simulink model "Single_Phase_Rectifier"  (R2023b)
settings: Solver=VariableStepAuto  StartTime=0.0  StopTime=0.1  MaxStep=2e-4  RelTol=1e-3
libraries: spsDetailedThyristorLib x4, spsACVoltageSourceLib x1, spsMultimeterLib x1, spsSeriesRLCBranchLib x1, sps_lib x1
settings Model: Creator=33034  LastModifiedBy=33034

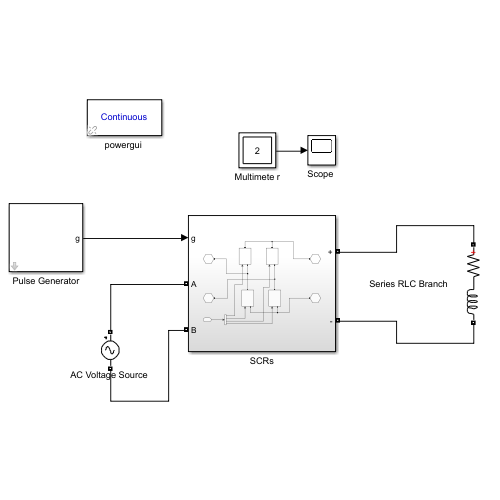
[thumbnail: Simulink's stored preview of the top-level diagram]
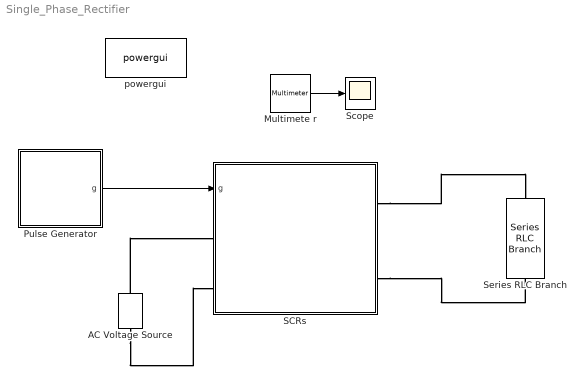
== system Single_Phase_Rectifier ==
  "AC Voltage Source " : spsACVoltageSourceLib/AC Voltage Source  Amplitude=220*sqrt(2)  Phase=0  Frequency=50  SampleTime=0  Measurements=None  BusType=swing  Pref=10e3  Qref=0  Qmin=-inf  Qmax=+inf
  Multimete r : spsMultimeterLib/Multimeter  L=2  sel=[1 2]  yselected={}  Gain=[1 1]  OutputType=Complex  PlotAtSimulationStop=off  PhasorSimulation=off
  Pulse Generator : Subsystem  mask{freq=50, alpha=90}
      mask prompts: freq "频率"
      mask DialogControl ParameterGroupVar Prompt: 参数
  SCRs : Subsystem
  "Scope " : Scope
  "Series RLC Branch " : spsSeriesRLCBranchLib/Series RLC Branch  LConnTagsString=__new0  RConnTagsString=__new0  BranchType=RL  Resistance=10  Inductance=1  SetiL0=off  InitialCurrent=0  Capacitance=1e-6  Setx0=off  InitialVoltage=0  Measurements=Branch voltage and current
  "powergui " : sps_lib/powergui  Priority=1  SimulationMode=Continuous  SampleTime=50e-6  frequency=60  Iterations=50  frequencyindice=50  Pbase=100e6  ErrMax=1e-4  UnitsV=kV  UnitsW=MW  buscounter=0  FunctionMessages=off  echomessages=off  EnableUseOfTLC=off  CurrentSourceSwitches=off  DisableSnubberDevices=off  DisableRonSwitches=off  DisableVfSwitches=off  DisplayEquations=off  AutomaticDiscreteSolvers=off  SolverType=Tustin/Backward Euler (TBE)  Interpol=off  ExternalGateDelay=off  methode=off  Ts=100  x0status=blocks  SPID=on  SwTol=0  HookPort=off  NonlinearTolerance=1e-4  nMaxIteration=100  ContinueOnMaxIteration=off  RestoreLinks=warning  ResistiveCurrentMeasurement=off  Frange=[0:2:500]  Ylog=off  Xlog=on  ShowGrid=off  save=off  variable=ZData  structure=0  ZoomFFT=off  StartTime=0.0  cycles=1  DisplayStyle=1  fundamental=60  FreqAxis=off  MaxFrequency=1000  frequencyindicesteady=1  RmsSteady=1  display=off
  wires:
  Multimete r/1 -> "Scope "/1
  Pulse Generator/1(g) -> SCRs/1(g)
  connections:
  SCRs/RConn1 -- "Series RLC Branch "/LConn1
  SCRs/RConn2 -- "Series RLC Branch "/RConn1
  "AC Voltage Source "/RConn1 -- SCRs/LConn1
  "AC Voltage Source "/LConn1 -- SCRs/LConn2

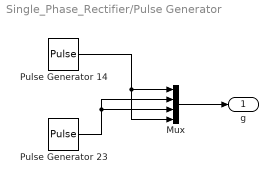
== system Single_Phase_Rectifier/Pulse Generator ==
  Mux : Mux
  Pulse Generator 14 : DiscretePulseGenerator  PulseType=Time based  Period=1/freq  PulseWidth=5  PhaseDelay=alpha/360*1/freq
  Pulse Generator 23 : DiscretePulseGenerator  PulseType=Time based  Period=1/freq  PulseWidth=5  PhaseDelay=(alpha+180)/360*1/freq
  g : Outport
  wires:
  Pulse Generator 14/1 -> Mux/4, Mux/1
  Pulse Generator 23/1 -> Mux/2, Mux/3
  Mux/1 -> g/1

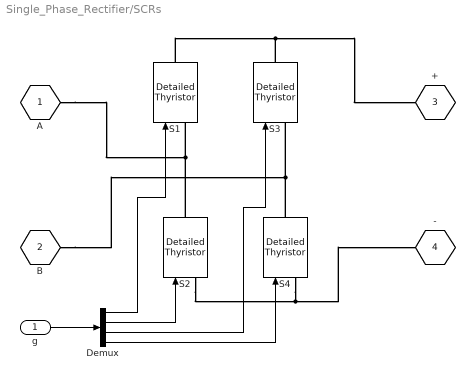
== system Single_Phase_Rectifier/SCRs ==
  g : Inport
  Demux : Demux
  S{1..4} (4 alike) : spsDetailedThyristorLib/Detailed Thyristor  Ron=0.001  Lon=1e-3  Vf=0.8  IL=0.1  Tq=100e-6  IC=0  Rs=500  Cs=250e-9  Measurements=off
      settings: LibrarySourceBlock=sps_lib/Power Electronics/Detailed Thyristor
  A : PMIOPort  Side=Left
  B : PMIOPort  Port=2  Side=Left
  + : PMIOPort  Port=3  Side=Right
  - : PMIOPort  Port=4  Side=Right
  wires:
  g/1 -> Demux/1
  Demux/1 -> S1/1
  Demux/2 -> S2/1
  Demux/3 -> S3/1
  Demux/4 -> S4/1
  connections:
  S4/RConn1 -- B/RConn1 -- S3/LConn1
  S2/RConn1 -- A/RConn1 -- S1/LConn1
  S1/RConn1 -- S3/RConn1 -- +/RConn1
  S2/LConn1 -- -/RConn1 -- S4/LConn1
